simulink model "clik_z_inverse"  (R2022b)
settings: Solver=ode1  StartTime=0.0  StopTime=4  FixedStep=0.001  RelTol=1e-3
undefined symbols (not defined in the file or in its folder): DiscIntNeverNeededParam, q0, Tc
settings Model: Creator=Xp  LastModifiedBy=anujs
settings SolverCC: AlgebraicLoopSolver=TrustRegion
settings DataIOCC: LimitDataPoints=on  SaveFormat=Array  SignalLoggingSaveFormat=ModelDataLogs  ReturnWorkspaceOutputs=off
settings OptimizationCC: ExpressionDepthLimit=2147483647  InitFltsAndDblsToZero=on  LifeSpan=inf
settings DebuggingCC: SaveWithParameterizedLinksMsg=none  UnderspecifiedInitializationDetection=Classic  MergeDetectMultiDrivingBlocksExec=none  SolverPrmCheckMsg=warning  MultiTaskDSMMsg=warning  MultiTaskCondExecSysMsg=none  FcnCallInpInsideContextMsg=warning  UnconnectedInputMsg=warning  UnconnectedOutputMsg=warning  UnconnectedLineMsg=warning  StateNameClashWarn=warning  SFUnexpectedBacktrackingDiag=warning  SFNoUnconditionalDefaultTransitionDiag=warning  SFExecutionAtInitializationDiag=none  SFMachineParentedDataDiag=warning  ArithmeticOperatorsInVariantConditions=warning
settings HardwareCC: ProdBitPerPointer=32  ProdBitPerSizeT=32  ProdBitPerPtrDiffT=32  ProdLargestAtomicFloat=None  ProdIntDivRoundTo=Undefined  ProdEndianess=Unspecified  ProdWordSize=32  ProdHWDeviceType=32-bit Generic
settings ModelReferenceCC: EnableRefExpFcnMdlSchedulingChecks=on  PropagateSignalLabelsOutOfModel=off
settings SFSimCC: CustomCodeUndefinedFunction=UseInterfaceOnly
settings RTWCC: DLArmComputeVersion=19.05
settings CodeAppCC: StateflowObjectComments=on
settings GRTTargetCC: TargetLangStandard=C89/C90 (ANSI)  CombineOutputUpdateFcns=off  GRTInterface=on
settings ConfigComp: CovMetricSettings=dw  CovSaveCumulativeToWorkspaceVar=on  CovSaveSingleToWorkspaceVar=on

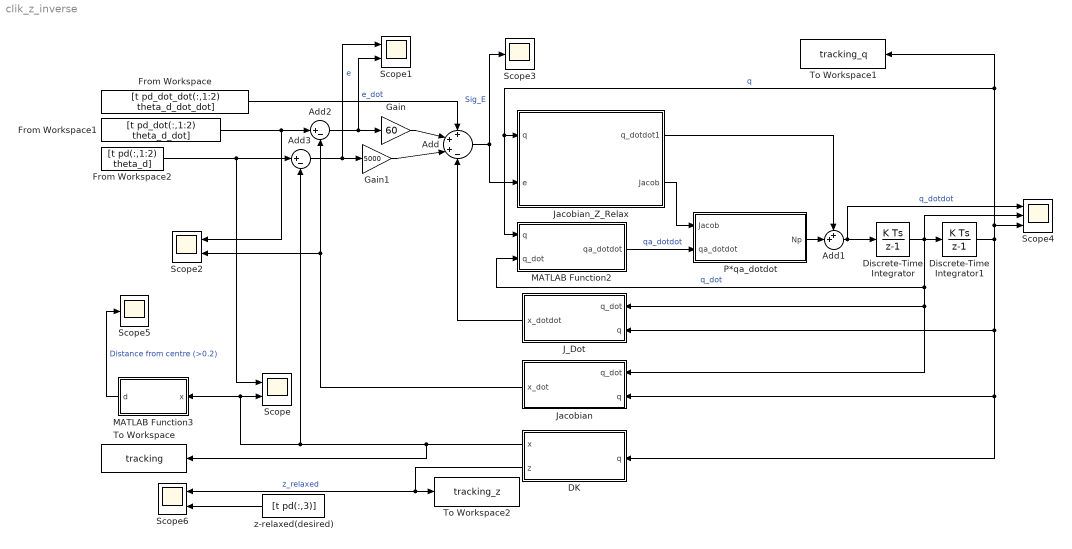
== system clik_z_inverse ==
  Add : Sum  Inputs=+++-
  Add1 : Sum  Inputs=++|
  Add2 : Sum  Inputs=|+-
  Add3 : Sum  Inputs=|+-
  DK : MATLAB Function  TreatAsAtomicUnit=on
  Discrete-Time Integrator : DiscreteIntegrator  InitialCondition=q0  SampleTime=Tc  LimitOutput=on  UpperSaturationLimit=[pi 3*pi/4 0.75 4*pi]'  LowerSaturationLimit=[-pi -3*pi/4 -0.75 -4*pi]'  ICPrevOutput=DiscIntNeverNeededParam  ICPrevScaledInput=DiscIntNeverNeededParam
  Discrete-Time Integrator1 : DiscreteIntegrator  InitialCondition=q0  SampleTime=Tc  LimitOutput=on  UpperSaturationLimit=[pi/2 pi/4 1 2*pi]'  LowerSaturationLimit=[-pi/2 -pi/2 .25 -2*pi]'  ICPrevOutput=DiscIntNeverNeededParam  ICPrevScaledInput=DiscIntNeverNeededParam
  From Workspace : FromWorkspace  VariableName=[t pd_dot_dot(:,1:2) theta_d_dot_dot]  SampleTime=Tc
  From Workspace1 : FromWorkspace  VariableName=[t pd_dot(:,1:2) theta_d_dot]  SampleTime=Tc
  From Workspace2 : FromWorkspace  VariableName=[t pd(:,1:2) theta_d]  SampleTime=Tc
  Gain : Gain  Gain=60
  Gain1 : Gain  Gain=5000
  J_Dot : MATLAB Function  TreatAsAtomicUnit=on
  Jacobian : MATLAB Function  TreatAsAtomicUnit=on
  Jacobian_Z_Relax : MATLAB Function  TreatAsAtomicUnit=on
  MATLAB Function2 : MATLAB Function  TreatAsAtomicUnit=on
  MATLAB Function3 : MATLAB Function  TreatAsAtomicUnit=on
  P*qa_dotdot : MATLAB Function  TreatAsAtomicUnit=on
  Scope{,1..2,6} (4 alike) : Scope  NumInputPorts=2
  Scope3 : Scope
  Scope4 : Scope  NumInputPorts=3
  Scope5 : Scope
  To Workspace : ToWorkspace  VariableName=tracking  SampleTime=Tc
  To Workspace1 : ToWorkspace  VariableName=tracking_q  SampleTime=Tc
  To Workspace2 : ToWorkspace  VariableName=tracking_z  SampleTime=Tc
  z-relaxed(desired) : FromWorkspace  VariableName=[t pd(:,3)]  OutDataTypeStr=double  SampleTime=Tc  OutputAfterFinalValue=Holding final value
  wires:
  J_Dot/1(x_dotdot) -> Add/4
  Gain/1 -> Add/2
  Gain1/1 -> Add/3
  From Workspace/1 -> Add/1
  Add/1 -> Jacobian_Z_Relax/2(e), Scope3/1  "Sig_E"
  Jacobian_Z_Relax/1(q_dotdot1) -> Add1/1
  P*qa_dotdot/1(Np) -> Add1/2
  Add2/1 -> Scope1/2, Gain/1  "e_dot"
  Add3/1 -> Scope1/1, Gain1/1  "e"
  Add1/1 -> Discrete-Time Integrator/1, Scope4/1  "q_dotdot"
  Discrete-Time Integrator1/1 -> To Workspace1/1, MATLAB Function2/1(q), Jacobian_Z_Relax/1(q), Scope4/3, J_Dot/2(q), DK/1(q), Jacobian/2(q)  "q"
  Jacobian_Z_Relax/2(Jacob) -> P*qa_dotdot/1(Jacob)
  MATLAB Function2/1(qa_dotdot) -> P*qa_dotdot/2(qa_dotdot)  "qa_dotdot"
  Jacobian/1(x_dot) -> Add2/2, Scope2/2
  DK/1(x) -> To Workspace/1, Add3/2, Scope/2, MATLAB Function3/1(x)
  From Workspace2/1 -> Add3/1, Scope/1
  From Workspace1/1 -> Scope2/1, Add2/1
  MATLAB Function3/1(d) -> Scope5/1  "Distance from centre (>0.2)"
  DK/2(z) -> To Workspace2/1, Scope6/1  "z_relaxed"
  z-relaxed(desired)/1 -> Scope6/2
  Discrete-Time Integrator/1 -> Discrete-Time Integrator1/1, Scope4/2, MATLAB Function2/2(q_dot), J_Dot/1(q_dot), Jacobian/1(q_dot)  "q_dot"

== matlab function clik_z_inverse/Jacobian_Z_Relax ==
  data: q input; q_dotdot1 output; Jacob output; e input
function [q_dotdot1,Jacob] = Jacobian_PseudoInverse(q, e)

[q_dotdot1,Jacob] = jacobian_z_relax(q, e);
end

== matlab function clik_z_inverse/J_Dot ==
  data: q_dot input; x_dotdot output; q input
function x_dotdot = Jacobain_dot(q_dot, q)

x_dotdot = jacobian_dot(q_dot, q);
end

== matlab function clik_z_inverse/P*qa_dotdot ==
  data: Jacob input; Np output; qa_dotdot input
function Np = fcn(Jacob,qa_dotdot)




Np = (eye(4) - (pinv(Jacob))*Jacob)*qa_dotdot;

== matlab function clik_z_inverse/Jacobian ==
  data: q_dot input; x_dot output; q input
function x_dot = Jacob(q_dot, q)

%Link length
a1 = 0.5;
a2 = 0.5;

%Joint Variables
t1 = q(1);
t2 = q(2);
d3 = q(3);
t4 = q(4);


Ab0 = [1 0 0 0;0 1 0 0;0 0 1 1;0 0 0 1];
A01 = [cos(t1) -sin(t1) 0 a1*cos(t1); sin(t1) cos(t1) 0 a1*sin(t1); 0 0 1 0; 0 0 0 1];
A12 = [cos(t2) -sin(t2) 0 a2*cos(t2); sin(t2) cos(t2) 0 a2*sin(t2);0 0 1 0;0 0 0 1];
A23 = [1 0 0 0;0 1 0 0;0 0 1 -d3;0 0 0 1];
A34 = [cos(t4) -sin(t4) 0 0;sin(t4) cos(t4) 0 0;0 0 1 0;0 0 0 1];

Ab1 = Ab0*A01;
Ab2 = Ab1*A12;
Ab3 = Ab2*A23;
Ab4 = Ab3*A34;

z0 = [0 0 1]';
z1 = [0 0 1]';
z2 = [0 0 1]';
z3 = [0 0 1]';
z4 = [0 0 1]';

J_1 = cross(z0,Ab4(1:3,4));
J_2 = cross(z1,(Ab4(1:3,4) - Ab1(1:3,4)));
J_4 = cross(z3,(Ab4(1:3,4) - Ab3(1:3,4)));



jac = [[J_1 J_2 z2 J_4];[z0 z1 [0 0 0]' z3]];
Jacobian = ([jac(1:2,:); jac(end,:)]);


x_dot = Jacobian*q_dot;

== matlab function clik_z_inverse/DK ==
  data: q input; x output; z output
function [x,z]= fcn(q)
%#codegen

[x,z] = direct_kin(q);

== matlab function clik_z_inverse/MATLAB Function2 ==
  data: q input; qa_dotdot output; q_dot input
function qa_dotdot = RedVect(q, q_dot)

t1=q(1);
t2=q(2);
d3=q(3);

ka = 3;


t1_dot=q_dot(1);
t2_dot=q_dot(2);
d3_dot=q_dot(3);


qa_dotdot = ka.*[(((2*(sin(t1)/2 + sin(t1 + t2)/2)*(cos(t1)/2 + cos(t1 + t2)/2 - 2/5)^2)/((cos(t1)/2 + cos(t1 + t2)/2 - 2/5)^2)^(1/2) - (2*(cos(t1)/2 + cos(t1 + t2)/2)*(sin(t1)/2 + sin(t1 + t2)/2 + 7/10)^2)/((sin(t1)/2 + sin(t1 + t2)/2 + 7/10)^2)^(1/2))*(2*((cos(t1)*t1_dot)/2 + (cos(t1 + t2)*(t1_dot + t2_dot))/2)*(sin(t1)/2 + sin(t1 + t2)/2 + 7/10) - 2*((sin(t1)*t1_dot)/2 + (sin(t1 + t2)*(t1_dot + t2_dot))/2)*(cos(t1)/2 + cos(t1 + t2)/2 - 2/5) + 2*(d3 - 129/500)*d3_dot))/(4*((cos(t1)/2 + cos(t1 + t2)/2 - 2/5)^2 + (sin(t1)/2 + sin(t1 + t2)/2 + 7/10)^2 + (d3 - 129/500)^2)^(3/2)) - ((2*((cos(t1)*t1_dot)/2 + (cos(t1 + t2)*(t1_dot + t2_dot))/2)*(cos(t1)/2 + cos(t1 + t2)/2 - 2/5)^2)/((cos(t1)/2 + cos(t1 + t2)/2 - 2/5)^2)^(1/2) + (2*((sin(t1)*t1_dot)/2 + (sin(t1 + t2)*(t1_dot + t2_dot))/2)*(sin(t1)/2 + sin(t1 + t2)/2 + 7/10)^2)/((sin(t1)/2 + sin(t1 + t2)/2 + 7/10)^2)^(1/2) + (2*(sin(t1)/2 + sin(t1 + t2)/2)*((sin(t1)*t1_dot)/2 + (sin(t1 + t2)*(t1_dot + t2_dot))/2)*(cos(t1)/2 + cos(t1 + t2)/2 - 2/5)^3)/((cos(t1)/2 + cos(t1 + t2)/2 - 2/5)^2)^(3/2) + (2*((cos(t1)*t1_dot)/2 + (cos(t1 + t2)*(t1_dot + t2_dot))/2)*(cos(t1)/2 + cos(t1 + t2)/2)*(sin(t1)/2 + sin(t1 + t2)/2 + 7/10)^3)/((sin(t1)/2 + sin(t1 + t2)/2 + 7/10)^2)^(3/2) - (4*(sin(t1)/2 + sin(t1 + t2)/2)*((sin(t1)*t1_dot)/2 + (sin(t1 + t2)*(t1_dot + t2_dot))/2)*(cos(t1)/2 + cos(t1 + t2)/2 - 2/5))/((cos(t1)/2 + cos(t1 + t2)/2 - 2/5)^2)^(1/2) - (4*((cos(t1)*t1_dot)/2 + (cos(t1 + t2)*(t1_dot + t2_dot))/2)*(cos(t1)/2 + cos(t1 + t2)/2)*(sin(t1)/2 + sin(t1 + t2)/2 + 7/10))/((sin(t1)/2 + sin(t1 + t2)/2 + 7/10)^2)^(1/2))/(2*((cos(t1)/2 + cos(t1 + t2)/2 - 2/5)^2 + (sin(t1)/2 + sin(t1 + t2)/2 + 7/10)^2 + (d3 - 129/500)^2)^(1/2));...
(((sin(t1 + t2)*(cos(t1)/2 + cos(t1 + t2)/2 - 2/5)^2)/((cos(t1)/2 + cos(t1 + t2)/2 - 2/5)^2)^(1/2) - (cos(t1 + t2)*(sin(t1)/2 + sin(t1 + t2)/2 + 7/10)^2)/((sin(t1)/2 + sin(t1 + t2)/2 + 7/10)^2)^(1/2))*(2*((cos(t1)*t1_dot)/2 + (cos(t1 + t2)*(t1_dot + t2_dot))/2)*(sin(t1)/2 + sin(t1 + t2)/2 + 7/10) - 2*((sin(t1)*t1_dot)/2 + (sin(t1 + t2)*(t1_dot + t2_dot))/2)*(cos(t1)/2 + cos(t1 + t2)/2 - 2/5) + 2*(d3 - 129/500)*d3_dot))/(4*((cos(t1)/2 + cos(t1 + t2)/2 - 2/5)^2 + (sin(t1)/2 + sin(t1 + t2)/2 + 7/10)^2 + (d3 - 129/500)^2)^(3/2)) - ((sin(t1 + t2)*(t1_dot + t2_dot)*(sin(t1)/2 + sin(t1 + t2)/2 + 7/10)^2)/((sin(t1)/2 + sin(t1 + t2)/2 + 7/10)^2)^(1/2) - (2*sin(t1 + t2)*((sin(t1)*t1_dot)/2 + (sin(t1 + t2)*(t1_dot + t2_dot))/2)*(cos(t1)/2 + cos(t1 + t2)/2 - 2/5))/((cos(t1)/2 + cos(t1 + t2)/2 - 2/5)^2)^(1/2) - (2*cos(t1 + t2)*((cos(t1)*t1_dot)/2 + (cos(t1 + t2)*(t1_dot + t2_dot))/2)*(sin(t1)/2 + sin(t1 + t2)/2 + 7/10))/((sin(t1)/2 + sin(t1 + t2)/2 + 7/10)^2)^(1/2) + (sin(t1 + t2)*((sin(t1)*t1_dot)/2 + (sin(t1 + t2)*(t1_dot + t2_dot))/2)*(cos(t1)/2 + cos(t1 + t2)/2 - 2/5)^3)/((cos(t1)/2 + cos(t1 + t2)/2 - 2/5)^2)^(3/2) + (cos(t1 + t2)*((cos(t1)*t1_dot)/2 + (cos(t1 + t2)*(t1_dot + t2_dot))/2)*(sin(t1)/2 + sin(t1 + t2)/2 + 7/10)^3)/((sin(t1)/2 + sin(t1 + t2)/2 + 7/10)^2)^(3/2) + (cos(t1 + t2)*(t1_dot + t2_dot)*(cos(t1)/2 + cos(t1 + t2)/2 - 2/5)^2)/((cos(t1)/2 + cos(t1 + t2)/2 - 2/5)^2)^(1/2))/(2*((cos(t1)/2 + cos(t1 + t2)/2 - 2/5)^2 + (sin(t1)/2 + sin(t1 + t2)/2 + 7/10)^2 + (d3 - 129/500)^2)^(1/2));...
(12500*(500*d3 - 129)^3*(5000*cos(t2)*d3_dot + 903*cos(t1)*t1_dot + 516*sin(t1)*t1_dot - 645*sin(t2)*t2_dot + 11500*d3_dot + 903*cos(t1 + t2)*t1_dot + 903*cos(t1 + t2)*t2_dot + 516*sin(t1 + t2)*t1_dot + 516*sin(t1 + t2)*t2_dot - 3500*cos(t1)*d3*t1_dot - 2000*sin(t1)*d3*t1_dot + 2500*sin(t2)*d3*t2_dot - 1000*65^(1/2)*cos(atan(7/4) + t1 + t2)*d3_dot - 1000*65^(1/2)*cos(atan(7/4) + t1)*d3_dot - 3500*cos(t1 + t2)*d3*t1_dot - 3500*cos(t1 + t2)*d3*t2_dot - 2000*sin(t1 + t2)*d3*t1_dot - 2000*sin(t1 + t2)*d3*t2_dot))/(((500*d3 - 129)^2)^(3/2)*(125000*cos(t2) - 129000*d3 + 250000*d3^2 - 25000*65^(1/2)*cos(atan(7/4) + t1 + t2) - 25000*65^(1/2)*cos(atan(7/4) + t1) + 304141)^(3/2));...
0];

end

== matlab function clik_z_inverse/MATLAB Function3 ==
  data: x input; d output
function d = dist_check(x)

t1 = x(1);
t2 = x(2);
d3 = x(3);






d = ((t1-0.4)^2 + (t2+0.7)^2 + (d3-0.5)^2)^0.5;
